simulink model "simmodel_24"  (R2024a)
settings: Solver=ode45  StartTime=0.0  StopTime=150  RelTol=1e-9  EnableMultiTasking=on
values from neighbouring files (symbols this model uses):
  K = 3.86    [Copy_of_benchmark.m]    (also in benchmark.m = 17.85; setpidparam.m)
  mu = 0.1    [Copy_of_benchmark.m]    (also in benchmark.m; setpidparam.m)
  N = 4    [Copy_of_benchmark.m]    (also in benchmark.m = 2; setpidparam.m = 3)
  Td = 0    [Copy_of_benchmark.m]    (also in benchmark.m = 0.2983; setpidparam.m)
  theta = [anti_wind_up; anti_bump; Kf]    [Copy_of_benchmark.m]    (also in benchmark.m = [0]; setpidparam.m = [1; 1; Kf; u0])
  Ti = 27    [Copy_of_benchmark.m]    (also in benchmark.m = 1.1932; setpidparam.m)
  Ts = 0.02    [Copy_of_benchmark.m]    (also in benchmark.m; setpidparam.m)
  ubounds = [0;10]    [Copy_of_benchmark.m]    (also in benchmark.m = [-6;6]; setpidparam.m)
libraries: cstblocks x2
settings Model: Creator=petersson  LastModifiedBy=ollha403
settings SolverCC: AlgebraicLoopSolver=TrustRegion
settings DataIOCC: LimitDataPoints=on  SaveFormat=Array  SignalLoggingSaveFormat=ModelDataLogs  ReturnWorkspaceOutputs=off
settings OptimizationCC: ExpressionDepthLimit=2147483647  LifeSpan=inf
settings DebuggingCC: UnderspecifiedInitializationDetection=Classic  MergeDetectMultiDrivingBlocksExec=none  SolverPrmCheckMsg=warning  FcnCallInpInsideContextMsg=warning  UnconnectedInputMsg=warning  UnconnectedOutputMsg=warning  UnconnectedLineMsg=warning  StateNameClashWarn=warning  SFUnexpectedBacktrackingDiag=warning  SFNoUnconditionalDefaultTransitionDiag=warning  SFExecutionAtInitializationDiag=none  ArithmeticOperatorsInVariantConditions=warning
settings HardwareCC: ProdBitPerPointer=32  ProdBitPerSizeT=32  ProdBitPerPtrDiffT=32  ProdLargestAtomicFloat=None  ProdIntDivRoundTo=Undefined  ProdEndianess=Unspecified  ProdWordSize=32  ProdHWDeviceType=32-bit Generic
settings ModelReferenceCC: PropagateSignalLabelsOutOfModel=off
settings SFSimCC: SimUseLocalCustomCode=off  SimParseCustomCode=off  CustomCodeUndefinedFunction=UseInterfaceOnly
settings RTWCC: RTWUseLocalCustomCode=off  GPUComputeCapability=3.5
settings CodeAppCC: StateflowObjectComments=on
settings GRTTargetCC: TargetLangStandard=C89/C90 (ANSI)  CombineOutputUpdateFcns=off  GRTInterface=on
settings ConfigComp: CovMetricSettings=dw  CovSaveCumulativeToWorkspaceVar=on  CovSaveSingleToWorkspaceVar=on  CovExternalEMLEnable=off

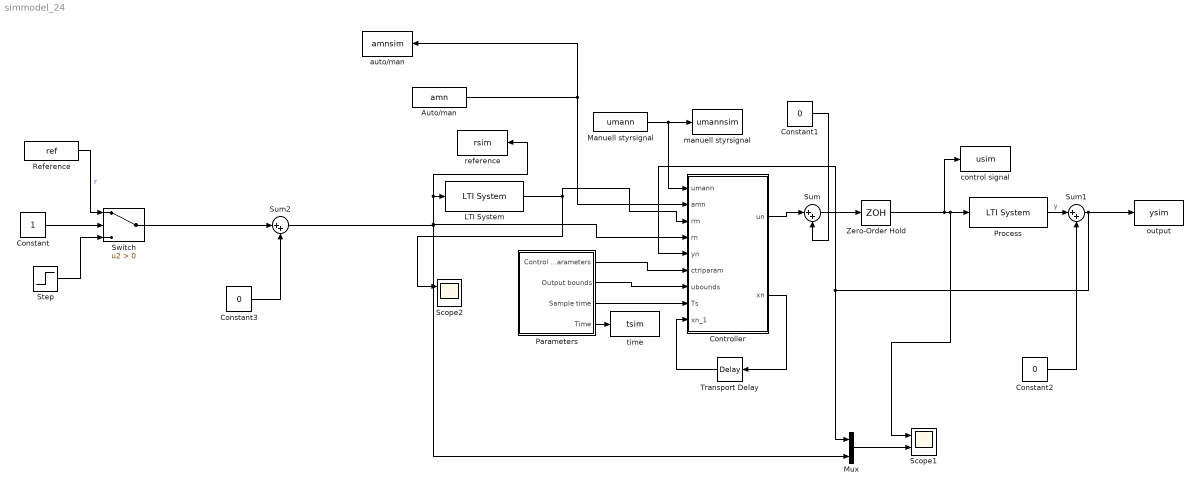
== system simmodel_24 ==
  Auto/man : FromWorkspace  VariableName=amn  SampleTime=Ts
  Constant : Constant
  Constant1 : Constant  Value=0
  Constant2 : Constant  Value=0
  Constant3 : Constant  Value=0
  Controller : MATLAB Function  TreatAsAtomicUnit=on
  LTI System : cstblocks/LTI System  sys=Gm  IC=[]  PadeOrder=0
  Manuell styrsignal : FromWorkspace  VariableName=umann  SampleTime=Ts
  Mux : Mux  Inputs=2
  Parameters : Subsystem
  Process : cstblocks/LTI System  sys=sys  IC=[]  PadeOrder=0
  Reference : FromWorkspace  VariableName=ref  SampleTime=Ts
  Scope1 : Scope  NumInputPorts=2
  Scope2 : Scope  NumInputPorts=2
  Step : Step  SampleTime=0
  Sum : Sum  Inputs=|++
  Sum1 : Sum  Inputs=|++
  Sum2 : Sum  Inputs=|++
  Switch : Switch  Criteria=u2 > Threshold  SaturateOnIntegerOverflow=off  InputSameDT=off
  Transport Delay : TransportDelay  DelayTime=Ts  InitialOutput=zeros(N,1)  FixedBuffer=on
  Zero-Order Hold : ZeroOrderHold  SampleTime=Ts
  auto/man : ToWorkspace  VariableName=amnsim  SampleTime=Ts
  control signal : ToWorkspace  VariableName=usim  SampleTime=Ts
  manuell styrsignal : ToWorkspace  VariableName=umannsim  SampleTime=Ts
  output : ToWorkspace  VariableName=ysim  SampleTime=Ts
  reference : ToWorkspace  VariableName=rsim  SampleTime=Ts
  time : ToWorkspace  VariableName=tsim  SampleTime=Ts
  wires:
  Controller/2(xn) -> Transport Delay/1
  Transport Delay/1 -> Controller/9(xn_1)
  Parameters/1(Control parameters) -> Controller/6(ctrlparam)
  Parameters/2(Output bounds) -> Controller/7(ubounds)
  Parameters/3(Sample time) -> Controller/8(Ts)
  Parameters/4(Time) -> time/1
  Zero-Order Hold/1 -> Process/1, Scope1/1, control signal/1
  Manuell styrsignal/1 -> Controller/1(umann), manuell styrsignal/1
  Auto/man/1 -> Controller/2(amn), auto/man/1
  Mux/1 -> Scope1/2
  LTI System/1 -> Scope2/1, Controller/3(rm)
  Switch/1 -> Sum2/1
  Reference/1 -> Switch/1  "r"
  Step/1 -> Switch/3
  Constant/1 -> Switch/2
  Sum/1 -> Zero-Order Hold/1
  Controller/1(un) -> Sum/1
  Process/1 -> Sum1/1  "y"
  Sum1/1 -> Controller/5(yn), Mux/1, output/1
  Constant1/1 -> Sum/2
  Constant2/1 -> Sum1/2
  Sum2/1 -> reference/1, LTI System/1, Controller/4(rn), Mux/2
  Constant3/1 -> Sum2/2

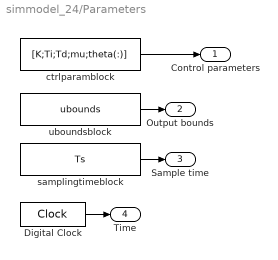
== system simmodel_24/Parameters ==
  Digital Clock : DigitalClock  SampleTime=Ts
  ctrlparamblock : Constant  Value=[K;Ti;Td;mu;theta(:)]
  samplingtimeblock : Constant  Value=Ts
  uboundsblock : Constant  Value=ubounds
  Control parameters : Outport
  Output bounds : Outport  Port=2
  Sample time : Outport  Port=3
  Time : Outport  Port=4
  wires:
  ctrlparamblock/1 -> Control parameters/1
  uboundsblock/1 -> Output bounds/1
  samplingtimeblock/1 -> Sample time/1
  Digital Clock/1 -> Time/1

== matlab function simmodel_24/Controller ==
  data: umann input; un output; amn input; rm input; rn input; yn input; ctrlparam input; ubounds input; Ts input; xn_1 input; xn output
function [un,xn]=computeux(umann,amn,rm,rn,yn,ctrlparam,ubounds,Ts,xn_1)
% STATE (N = 3):
%   xn_1(1) = I_mem   (integrator-minne FÖRE uppdatering)
%   xn_1(2) = e_prev  (föregående fel)
%   xn_1(3) = bias    (manual-bias för stötfri auto<->man)
%   xn_1(4) = D_mem

K     = double(ctrlparam(1));
Ti    = double(ctrlparam(2));
Td    = double(ctrlparam(3));
Mu    = double(ctrlparam(4));

theta = double(ctrlparam(5:end));   % ctrlparam = [K;Ti;Td;mu;Kf;theta(:)]

enableAW   = (numel(theta) >= 1) && (theta(1) ~= 0);
enableBump = (numel(theta) >= 2) && (theta(2) ~= 0);
Kf = theta(3);


% Cast inputs
umann = double(umann);
amn   = double(amn);
rn    = double(rn);
yn    = double(yn);
Ts    = double(Ts);

umin = double(ubounds(1));
umax = double(ubounds(2));

% Unpack state
I_mem  = double(xn_1(1));
e_prev = double(xn_1(2));
bias   = double(xn_1(3));
D_mem  = 0;
if numel(xn_1) >= 4
    D_mem = double(xn_1(4));
end

% Signals
e = rm - yn;

% Derivata (bakåtdifferens på felet)
if Td > 0
    Tf = Mu*Td; % filtertidkonstant
    if Tf > 0
        alpha = Tf/(Tf + Ts);
        D_mem = alpha*D_mem + (K*Td)/(Tf + Ts) * (e - e_prev);
        D = D_mem;
    else
        D = K * Td(e - e_prev)/Ts;
        D_mem = D;
    end
else
    D = 0;
    D_mem = 0;
end
P = K*e;

isAuto = (amn >= 0.5);   % 1=auto, 0=manuell

if isAuto
    % ===== AUTOMATISK MOD =====
    % Integrera (kandidat)
    I_cand = I_mem;
    if Ti > 0
        I_cand = I_mem + K*Ts*e/Ti;
    end

    % Kandidat-utgång före mättnad
    v_cand = P + I_cand + D;

    % Mättnad
    un = v_cand;
    un = un + rn*Kf;  %framkoppling och u0
    
    if un < umin, un = umin; end
    if un > umax, un = umax; end
    
    % Anti-windup (clamping): frys integrator om mättad och felet driver mer in i mättnad
    if enableAW && Ti > 0
        satHigh = (v_cand > umax) && (un >= umax);
        satLow  = (v_cand < umin) && (un <= umin);

        if (satHigh && e > 0) || (satLow && e < 0)
            % Frys integrator (revertera integration)
            I_cand = I_mem;

            % Räkna om med fryst integrator (kan av-mätta)
            v = P + I_cand + D;
            un = v;
            if un < umin, un = umin; end
            if un > umax, un = umax; end
        end
        
    end

    % Stötfri auto->man: uppdatera bias så att u = umann + bias blir kontinuerlig vid modbyte
    if enableBump
        bias = un - umann;
    else
        bias = 0;
    end

    % Spara integrator
    I_mem = I_cand;

else
    % ===== MANUELL MOD =====
    if enableBump
        % Stötfri: applicera manuellsignal med bias (bias hålls konstant i manuell mod)
        un = umann + bias;
    else
        % Icke-stötfri: ren manuell
        un = umann;
        bias = 0;
    end

    % Mättnad även i manuell mod
    if un < umin, un = umin; end
    if un > umax, un = umax; end

    % Stötfri man->auto: välj I_mem så att nästa autosampling ger v == un
    % Auto gör: I_cand = I_mem + K*Ts*e/Ti, v = P + I_cand + D.
    % Vill: v == un  => I_mem = un - P - D - K*Ts*e/Ti
    if enableBump && Ti > 0
        I_mem = un - P - D - K*Ts*e/Ti;
    end
end

% Pack next state
xn = [I_mem; e; bias; D_mem];
